simulink library "Power_Alpha"  (R2019b)
settings: Solver=ode45  StartTime=0.0  StopTime=10.0  RelTol=1e-3  EnableMultiTasking=on
undefined symbols (not defined in the file): Power
libraries: simulink x1
settings Model: Creator=mbrauer  LastModifiedBy=bhisma
settings DataIOCC: LimitDataPoints=on  SaveFormat=Array  SignalLoggingSaveFormat=ModelDataLogs  ReturnWorkspaceOutputs=off
settings OptimizationCC: LifeSpan=inf
settings DebuggingCC: SolverPrmCheckMsg=warning  MultiTaskDSMMsg=warning  MultiTaskCondExecSysMsg=none  SFUnexpectedBacktrackingDiag=warning  SFNoUnconditionalDefaultTransitionDiag=warning  SFExecutionAtInitializationDiag=none  ArithmeticOperatorsInVariantConditions=warning
settings HardwareCC: ProdBitPerPointer=32  ProdBitPerSizeT=32  ProdBitPerPtrDiffT=32  ProdLargestAtomicFloat=None  ProdIntDivRoundTo=Undefined  ProdEndianess=Unspecified  ProdWordSize=32  ProdHWDeviceType=32-bit Generic
settings ModelReferenceCC: PropagateSignalLabelsOutOfModel=off
settings SFSimCC: SimUseLocalCustomCode=off  CustomCodeUndefinedFunction=UseInterfaceOnly
settings RTWCC: RTWUseLocalCustomCode=off
settings CodeAppCC: StateflowObjectComments=on
settings GRTTargetCC: TargetLangStandard=C89/C90 (ANSI)  GeneratePreprocessorConditionals=Disable all
settings ConfigComp: CovMetricSettings=dw  CovHtmlReporting=on  CovSaveCumulativeToWorkspaceVar=on  CovSaveSingleToWorkspaceVar=on  CovExternalEMLEnable=off  CovSFcnEnable=off

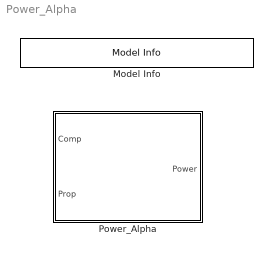
== system Power_Alpha ==
  Model Info : simulink/Model-Wide Utilities/Model Info  Frame=on  DisplayStringWithTags=Copyright 2013-2014 The MathWorks, Inc.  HorizontalTextAlignment=Center  LeftAlignmentValue=0.5
  Power_Alpha : Subsystem

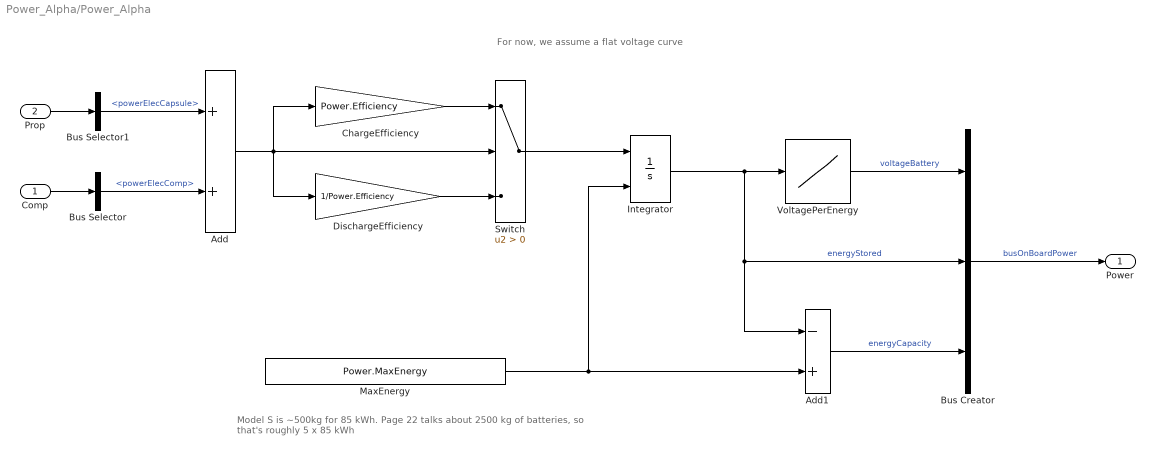
== system Power_Alpha/Power_Alpha ==
  note: Model S is ~500kg for 85 kWh.
      | Page 22 talks about 2500 kg of batteries, so that's roughly 5 x 85 kWh
  note: For now, we assume a flat voltage curve
  Comp : Inport
  Prop : Inport  Port=2
  Add : Sum
  Add1 : Sum  Inputs=-+
  Bus Creator : BusCreator  Inputs=3  NonVirtualBus=on
  Bus Selector : BusSelector  OutputSignals=powerElecComp
  Bus Selector1 : BusSelector  OutputSignals=powerElecCapsule
  ChargeEfficiency : Gain  Gain=Power.Efficiency
  DischargeEfficiency : Gain  Gain=1/Power.Efficiency
  Integrator : Integrator  InitialConditionSource=external
  MaxEnergy : Constant  Value=Power.MaxEnergy
  Switch : Switch  Criteria=u2 > Threshold
  VoltagePerEnergy : Lookup_n-D  NumberOfTableDimensions=1  BreakpointsForDimension1=[0 1e9]  Table=[600 600]  InternalRulePriority=Speed  RndMeth=Simplest  InputSameDT=on
  Power : Outport
  wires:
  Switch/1 -> Integrator/1
  DischargeEfficiency/1 -> Switch/3
  Add/1 -> ChargeEfficiency/1, Switch/2, DischargeEfficiency/1
  ChargeEfficiency/1 -> Switch/1
  Bus Selector1/1 -> Add/1  "<powerElecCapsule>"
  Integrator/1 -> VoltagePerEnergy/1, Add1/1, Bus Creator/2  "energyStored"
  Bus Creator/1 -> Power/1  "busOnBoardPower"
  MaxEnergy/1 -> Add1/2, Integrator/2
  Bus Selector/1 -> Add/2  "<powerElecComp>"
  Prop/1 -> Bus Selector1/1
  VoltagePerEnergy/1 -> Bus Creator/1  "voltageBattery"
  Add1/1 -> Bus Creator/3  "energyCapacity"
  Comp/1 -> Bus Selector/1
